simulink model "A1_Nonco_AM_SDR_skeleton"  (R2019b)
settings: Solver=VariableStepAuto  StartTime=0.0  StopTime=inf  RelTol=1e-3
libraries: dspmlti4 x1, sdrrlib x1, dspobslib x1
settings Model: Creator=mxian  LastModifiedBy=linesLK

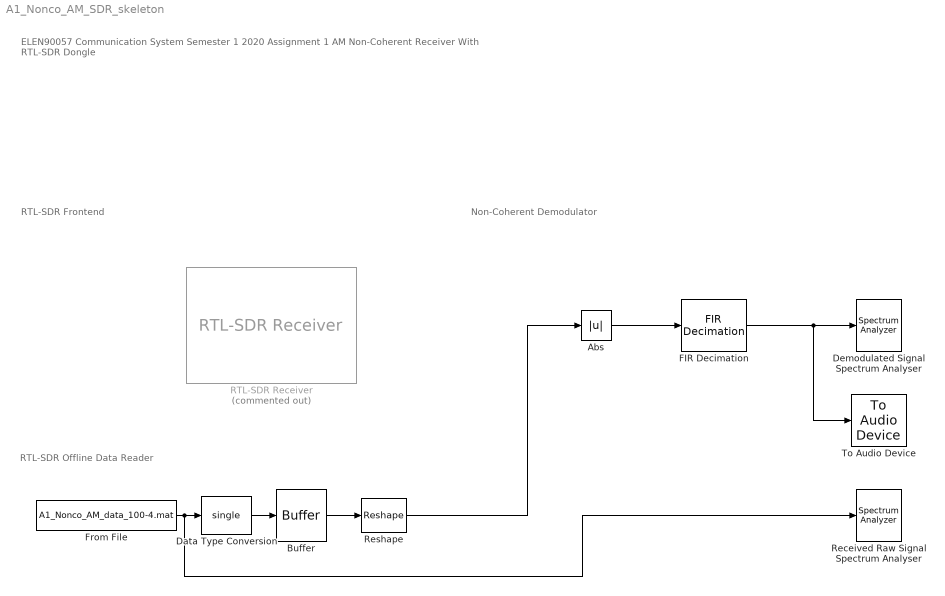
== system A1_Nonco_AM_SDR_skeleton ==
  note: ELEN90057 Communication System Semester 1 2020
      | Assignment 1
      | AM Non-Coherent Receiver With RTL-SDR Dongle
  note: RTL-SDR Frontend
  note: Non-Coherent Demodulator
  note: RTL-SDR Offline Data Reader
  Abs : Abs
  Buffer : Buffer  N=4096
  Data Type Conversion : DataTypeConversion  OutDataTypeStr=single
  Demodulated Signal Spectrum Analyser : SpectrumAnalyzer
  FIR Decimation : dspmlti4/FIR Decimation  FilterSource=Auto  h=firpm(100, [0 15e3 20e3 (240e3/2)]/(240e3/2), [1 1 0 0], [1 1], 20)  D=5  filtStruct=Direct form  FilterObject=Hm_firdecim  InputProcessing=Columns as channels (frame based)  framing=Allow multirate processing  inputOffset=0  outputBufInitCond=0  roundingMode=Floor  overflowMode=off  firstCoeffDataTypeStr=Inherit: Same word length as input  firstCoeffMin=[]  firstCoeffMax=[]  firstCoeffLastDataTypeStr=Inherit: Same word length as input  outputDataTypeStr=Inherit: Same as accumulator  outputMin=[]  outputMax=[]  outputLastDataTypeStr=Inherit: Same as accumulator
  "From File " : FromFile  FileName=A1_Nonco_AM_data_100-4.mat  OutDataTypeStr=single  SampleTime=4096/240e3  ExtrapolationAfterLastDataPoint=Ground value
  "RTL-SDR Receiver " : sdrrlib/RTL-SDR Receiver  Commented=on  IPAddress=0  CenterFrequencySource=Input port  CenterFrequency=89.8e6  GainSource=Input port  Gain=50  ADCRate=240e3  FrequencyCorrection=0  LostSamplesOutputPort=off  LatencyOutputPort=off  OutputDataType=single  FrameLength=4096  EnableBurstMode=off  NumFramesInBurst=20  sobjType=sdrr.internal.SDRRTLReceiverSL  dataUDPPort=-1  ctrlUDPPort=-1  subDeviceList=nosubdev  sdrBlockType=SDRBlockTypeSLT.SDRRxBlock  requester=UNUSED_BY_SFCN  sdrExecutionMode=SDRExecutionModeSLT.ExecModeHW  BypassUserLogic=off  DecimatorSelect=DDC decimator  SourceSelect=RF data  SineAmplitude=16000  EnableInternalClock=off  BypassIQBalance=off  IFBandwidth=40e6  ADCRateSource=Dialog  IntermediateFrequency=0  DecimationFactorSource=Dialog  DecimationFactor=512  RFFrequencyIsTunable=logical(1)  SampleTime=(4096)/(240e3)  IFBandwidthSource=Dialog  SineFrequency=30000  BypassDCBlockingFilter=off  IntermediateFrequencySource=Dialog  IQBalanceCoefficients=64  SkipAllHardwareResetAndInitialization=off  EnableIQCalibrationTable=on  CacheIQCalibrationTable=off  EnableOffsetTuning=off  EnableRTLAGC=off  EnableTestMode=off  EnableTunerAGC=off  FrequencyCorrectionSource=Dialog  NumMLBuffers=128  NumUSBBuffers=16  RTLCrystalFrequency=28800000  TunerCrystalFrequency=28800000
      settings: SourceProductName=Communications Toolbox Support Package for RTL-SDR Radio  SourceProductBaseCode=RTLSDR
  Received Raw Signal Spectrum Analyser : SpectrumAnalyzer
  Reshape : Reshape
  To Audio Device : dspobslib/To Audio Device  deviceName=Default  inheritSampleRate=on  sampleRate=44100  deviceDatatype=Determine from input data type  autoBufferSize=on  bufferSize=4096  queueDuration=1.0  defaultOutputChannelMapping=on  outputChannelMapping=1  outputNumUnderrunSamples=off
      settings: SourceProductName=DSP System Toolbox  SourceProductBaseCode=DS
  wires:
  Abs/1 -> FIR Decimation/1
  "From File "/1 -> Received Raw Signal Spectrum Analyser/1, Data Type Conversion/1
  Data Type Conversion/1 -> Buffer/1
  Buffer/1 -> Reshape/1
  Reshape/1 -> Abs/1
  FIR Decimation/1 -> To Audio Device/1, Demodulated Signal Spectrum Analyser/1
